simulink model "Gesamtmodell"  (R2017b)
settings: Solver=ode3  StartTime=0.0  StopTime=inf  FixedStep=dt  RelTol=1e-3  EnableMultiTasking=on
InitFcn:
  | Reglerauslegung
undefined symbols (not defined in the file or in its folder): aMax, aMaxPsi, Blindzeit, Com1, dt, K1, K2, K3, Kx, Ky, none, sigbuilder_block, Tx, Ty, vMax, vMaxPsi
libraries: xpcrtudplib x11, simulink x6, xpcutilitieslib x4, xpcseriallib x1, slrtlib x1
(part 3 of 4)

== matlab function Gesamtmodell/Regelung1/Receiver/autoRobID ==
  data: udpIn input; pX output; pY output; psi output; enable output; robID input
function [pX, pY, psi, enable] = autoRobID(udpIn, robID)
enable  = 1;
pX      = 0;
pY      = 0;
psi     = 0;

if robID == 1
    pX      = udpIn(1);
    pY      = udpIn(2);
    psi     = udpIn(3);
elseif robID == 2
    pX      = udpIn(4);
    pY      = udpIn(5);
    psi     = udpIn(6);
elseif robID == 3
    pX      = udpIn(7);
    pY      = udpIn(8);
    psi     = udpIn(9);
elseif robID == 4
    pX      = udpIn(10);
    pY      = udpIn(11);
    psi     = udpIn(12);
elseif robID == 5
    pX      = udpIn(13);
    pY      = udpIn(14);
    psi     = udpIn(15);
end

if (pX == 0) && (pY == 0)
    enable = 0;
end

== matlab function Gesamtmodell/Regelung1/Receiver/x4(psi) ==
  data: psi input; x4 output
function x4 = Winkelkorrektur(psi)

persistent turnCounter firstRun lastAngle

if isempty(firstRun)
    firstRun = 1;
    turnCounter = 0;
    lastAngle = 0;
end

% Kamera gibt uns -pi bis + pi
% Wir wollen 0 bis 2pi
psi = mod(psi+2*pi,2*pi);

% winkel kontinuierlich hoch bzw runterzaehlen
if( (psi < (2*pi)/5) && (lastAngle > ((2*pi) - (2*pi)/5) ) )
    turnCounter = turnCounter + 1;
end

if( (lastAngle < (2*pi)/5) && (psi > ((2*pi) - (2*pi)/5) ) )
    turnCounter = turnCounter - 1;
end

lastAngle = psi;

x4 = psi + turnCounter * 2*pi;

== matlab function Gesamtmodell/Regelung1/Robotino interface/assemble robotino response ==
  data: v_x_in input; robotino_response output; v_y_in input; v_theta_in input; distance_measuring_sensors_in input; bumper_in input; light_barrier_in input; slider_in input
%%%%%%%%%%%%%%%%%%%%%%%%%%%%%%%%%%%%%%%%%%%%%%%%%%%%%%%%%%%%%%%%%%%%%%%%%%%
% Assembly of robot data in a vector of 34 elements.                      %
%                                                                         %
% inputs:   longitudinal, lateral and rotational velocity (in mm/s),      %
%           shaft positions of the three motors (4 elements per motor),   %
%           running times of the three motors (3 elements per motor),     %
%           values of the nine IR-sensors (in mm),                        %
%           bumper collision (1 = no collision;                           %
%                             0 = collision)                              %
% outputs:  vector containing assembled input data                        %
%%%%%%%%%%%%%%%%%%%%%%%%%%%%%%%%%%%%%%%%%%%%%%%%%%%%%%%%%%%%%%%%%%%%%%%%%%%
function robotino_response = fcn(v_x_in, v_y_in, v_theta_in, ...
                                 distance_measuring_sensors_in, ...
                                 bumper_in, light_barrier_in, slider_in)
                                 % motor_positions_in, time_bytes_in, ...)
robotino_response = [light_barrier_in, slider_in, v_x_in, v_y_in, ...
                     v_theta_in, ...%motor_positions_in, time_bytes_in, ...
                     distance_measuring_sensors_in, bumper_in]';

== matlab function Gesamtmodell/Regelung1/Robotino interface/distance converter ==
  settings: sampleTime=dtpc/2
  data: dms_in input; dms_out output
%%%%%%%%%%%%%%%%%%%%%%%%%%%%%%%%%%%%%%%%%%%%%%%%%%%%%%%%%%%%%%%%%%%%%%%%%%%
% conversion of the nine distance measuring sensor values (resolution:    %
% 1Byte) to unit milimeters (range: from 40mm to 1500mm) with linear      %
% interpolation                                                           %
%                                                                         %
% input:  vector containing the values of the nine distance measuring     %
%         sensors                                                         %
% output: vector containing the nine values in milimeters                 %
%%%%%%%%%%%%%%%%%%%%%%%%%%%%%%%%%%%%%%%%%%%%%%%%%%%%%%%%%%%%%%%%%%%%%%%%%%%
function dms_out = fcn(dms_in)

y_mm = [40, 45, 50, 60, 75, 100, 125, 150, 175, 200, 250, 300]; % , ...
        %400, 500, 600, 700, 800, 900, 1000, 1100, 1200, 1300, 1500];
    
x_sensor = [255, 249.7733813, 228.6082474, 193.6871795, ...
            152.0044843, 113.7266187, 92.42268041, ...
            76.36407767, 65.19289827, 55.1025641, ...
            43.06299213, 34.97068404]; % , 24.37410072, ...
            % 16.3381295, 11.62589928, 8.661870504, ...
            % 6.316546763, 4.74, 3.65, 2.96, 2.40, ...
            % 2.035971223, 1.539568345];

% x_sensor = round(100 * x_sensor) / 100;

dms_out = interp1(x_sensor, y_mm, dms_in, 'linear');

== matlab function Gesamtmodell/Regelung1/Robotino interface/light barrier & slider ==
  data: di03_bump_in input; light_barrier output; slider output
function [light_barrier, slider] = fcn(di03_bump_in)
%%%%%%%%%%%%%%%%%%%%%%%%%%%%%%%%%%%%%%%%%%%%%%%%%%%%%%%%%%%%%%%%%%%%%%%%%%%
% di03_bump_in = 0 alternatively 12 ->  no light barrier activation       %
%                                       no slider activation              %
% di03_bump_in = 13                 ->  only light barrier activation     %
% di03_bump_in = 14                 ->  only slider activation            %
% di03_bump_in = 15                 ->  light barrier activation          %
%                                       slider activation                 %
%%%%%%%%%%%%%%%%%%%%%%%%%%%%%%%%%%%%%%%%%%%%%%%%%%%%%%%%%%%%%%%%%%%%%%%%%%%
% function [light_barrier, slider] = fcn(di03_bump_in)
% bin = dec2bin(di03_bump_in);
% if bin(3) == 1
%     light_barrier = 1;
% else
%     light_barrier = 0;
% end
% if bin(4) == 1
%     slider = 1;
% else
%     slider = 0;
% end
if     di03_bump_in == 13
    light_barrier = 1;
    slider        = 0;
elseif di03_bump_in == 14
    light_barrier = 0;
    slider        = 1;
elseif di03_bump_in == 15
    light_barrier = 1;
    slider        = 1;
else
    light_barrier = 0;
    slider        = 0;
end

== matlab function Gesamtmodell/Regelung1/Robotino interface/receive direction, unit & velocity converter ==
  settings: sampleTime=dtpc/2
  data: number_of_robot input; direction_motor0_in input; v_x_out output; velocity_motor0_in input; direction_motor1_in input; velocity_motor1_in input; direction_motor2_in input; velocity_motor2_in input; v_y_out output; v_theta_out output
%%%%%%%%%%%%%%%%%%%%%%%%%%%%%%%%%%%%%%%%%%%%%%%%%%%%%%%%%%%%%%%%%%%%%%%%%%%
% assembly of the three separate positive motor velocities (resolution:   %
% 1Byte) and their rotation direction to positive and/or negative         %
% longitudinal, lateral & rotational velocities (in milimeters per        %
% second)                                                                 %
%                                                                         %
% inputs:  direction_motor0_in (rotating direction of motor0              %
%          (129 := counter-clockwise; 128 := clockwise)),                 %
%          velocity_motor0_in (from 0 to 255),                            %
%          direction_motor1_in (rotating direction of motor1              %
%          (0 := counter-clockwise; 1 := clockwise)),                     %
%          velocity_motor1_in (from 0 to 255),                            %
%          direction_motor2_in (rotating direction of motor2              %
%          (0 := counter-clockwise; 1 := clockwise)),                     %
%          velocity_motor2_in (from 0 to 255)                             %
% outputs: v_x_out (longitudinal velocity (in milimeters per second)),    %
%          v_y_out (lateral velocity (in milimeters per second)),         %
%          v_theta_out (rotational velocity (in milimeters per second))   %
%%%%%%%%%%%%%%%%%%%%%%%%%%%%%%%%%%%%%%%%%%%%%%%%%%%%%%%%%%%%%%%%%%%%%%%%%%%
function [v_x_out, v_y_out, v_theta_out] ...
    = fcn(number_of_robot, direction_motor0_in, velocity_motor0_in, direction_motor1_in, ...
          velocity_motor1_in, direction_motor2_in, velocity_motor2_in)
%%%%%%%%%%%%%%%%%%%%%%%%%%%%%%%%%%%%%%%%%%%%%%%%%%%%%%%%%%%%%%%%%
% assembly of absolute motor velocity and rotating direction to %
% longitudinal, lateral & rotational velocity for every motor   %
%%%%%%%%%%%%%%%%%%%%%%%%%%%%%%%%%%%%%%%%%%%%%%%%%%%%%%%%%%%%%%%%%


% the direction bit for the motor 0 of robotino 3 is located at a different position
if number_of_robot == 3
    cmp = 1;
else
    cmp = 129;
end
    

if direction_motor0_in < cmp
    v0 = -velocity_motor0_in;
else
    v0 =  velocity_motor0_in;
end

if direction_motor1_in < 1
    v1 = -velocity_motor1_in;
else
    v1 =  velocity_motor1_in;
end

if direction_motor2_in < 1
    v2 = -velocity_motor2_in;
else
    v2 =  velocity_motor2_in;
end

%%%%%%%%%%%%%%%%%%%%%%%%%%%%%%%%%%%%%%%%%%%%%%%%%%%%%%%%%%%%%%%%%%%%%%%%%
% conversion of the separate motor velocities from a value between -255 %
% and 255 to millimeters                                                %
%%%%%%%%%%%%%%%%%%%%%%%%%%%%%%%%%%%%%%%%%%%%%%%%%%%%%%%%%%%%%%%%%%%%%%%%%
f_rcv = 7.02;
v0    = v0 * f_rcv;
v1    = v1 * f_rcv;
v2    = v2 * f_rcv;

%%%%%%%%%%%%%%%%%%%%%%%%%%%%%%%%%%%%%%%%%%%%%%%%%%%%%%%%%%%%%%%%%%%%
% conversion from three separate motor velocities to longitudinal, %
% lateral & rotational velocity                                    %
%%%%%%%%%%%%%%%%%%%%%%%%%%%%%%%%%%%%%%%%%%%%%%%%%%%%%%%%%%%%%%%%%%%%
v_x_out     = (v2 - v0) / (2 * cosd(30));                         % in mm/s
v_y_out     = (v0 - 2 * v1 + v2) / 3;                             % in mm/s
v_theta_out = (v0 + v1 + v2) / (3 * 135);                        % in rad/s

== matlab function Gesamtmodell/Regelung1/Robotino interface/serial communication/error filter & protocol disassembler ==
  settings: sampleTime=dtpc/2
  data: response input; error_free_resp_in input; direction_motor0_out output; velocity_motor0_out output; direction_motor1_out output; velocity_motor1_out output; direction_motor2_out output; velocity_motor2_out output; distance_measuring_sensors_out output; di03_bump_out output; bumper_out output; error_free_resp_out output
%%%%%%%%%%%%%%%%%%%%%%%%%%%%%%%%%%%%%%%%%%%%%%%%%%%%%%%%%%%%%%%%%%%%%%%%%%%
% Error check of the 'I/O-Board to PC104 message' and filtering of this   %
% defective response: Substitute defective message by the last error free %
% message.                                                                %
% Saving of the rotating direction, velocity, shaft position and running  %
% time of the three motors. Combining all shaft positions in a vector.    %
% Combining all running times in a vector.                                %
% Saving of the three bumper bytes indicating a collision in a vector.    %
% Saving the values of the nine distance measuring IR-sensors in a vector.%
%                                                                         %
% inputs: response (actual 'I/O-Board to PC104 message')(vector 102       %
%                   elements)                                             %
%         error_free_resp_in (last error free 'I/O-Board to PC104         %
%                             message')                                   %
% outputs: directions and velocities of the three motors                  %
%          motor_positions_out (shaft positions of the three motors)      %
%                              (vector 12 elements)                       %
%          time_bytes_out (running times of the three motors)             %
%                         (vector 9 elements)                             %
%          distance_measuring_sensors_out (values of the nine IR-sensors) %
%                                         (vector 9 elements)             %
%          bumper_out (vector 3 elements)                                 %
%          error_free_resp_out (error free 'I/O-Board to PC104 message')  %
%                              (vector 102 elements)                      %
%%%%%%%%%%%%%%%%%%%%%%%%%%%%%%%%%%%%%%%%%%%%%%%%%%%%%%%%%%%%%%%%%%%%%%%%%%%
function [direction_motor0_out, velocity_motor0_out, ...
          direction_motor1_out, velocity_motor1_out, ...
          direction_motor2_out, velocity_motor2_out, ...
          distance_measuring_sensors_out, di03_bump_out, bumper_out, ...
          error_free_resp_out] = fcn(response, error_free_resp_in)
%           motor_positions_out, time_bytes_out, ...)
      
%%%%%%%%%%%%%%%%%%%%%%%%%%%%%%%%%%%%%%%%%%%%%%%%%%%%%
% filtering defective 'I/O-Board to PC104 messages' %
%%%%%%%%%%%%%%%%%%%%%%%%%%%%%%%%%%%%%%%%%%%%%%%%%%%%%
if (response(1) == 101) && (response(2) == 82) && (response(3) == 69) ...
   && (response(4) == 67) && (response(100) == 114) ...        % if the ...
   && (response(101) == 101) && (response(102) == 99)  % counter (101), ...
                        % the start (REC) and stop (rec) bytes are true ...
    error_free_resp_out = response;     % save the actual 'I/O-Board to ...
                                                           % PC104 message'
else                                                        % otherwise ...
    error_free_resp_out = error_free_resp_in;     % save the last error ...
                                        % free 'I/O-Board to PC104 message'
end

%%%%%%%%%%%%%%%%%%%%%%%%%%%%%%%%%%%%%%%%%%%%%%%%%%%%%%%%%%%%%%%%%%%%%%%%%%
% save rotating direction, velocity, shaft position and the running time %
% of motor0                                                              %
%%%%%%%%%%%%%%%%%%%%%%%%%%%%%%%%%%%%%%%%%%%%%%%%%%%%%%%%%%%%%%%%%%%%%%%%%%
direction_motor0_out  = error_free_resp_out(26);
velocity_motor0_out   = error_free_resp_out(27);
% position_motor0_byte1 = error_free_resp_out(28);
% position_motor0_byte2 = error_free_resp_out(29);
% position_motor0_byte3 = error_free_resp_out(30);
% position_motor0_byte4 = error_free_resp_out(31);
% time_motor0_byte1     = error_free_resp_out(34);
% time_motor0_byte2     = error_free_resp_out(35);
% time_motor0_byte3     = error_free_resp_out(36);

%%%%%%%%%%%%%%%%%%%%%%%%%%%%%%%%%%%%%%%%%%%%%%%%%%%%%%%%%%%%%%%%%%%%%%%%%%
% save rotating direction, velocity, shaft position and the running time %
% of motor1                                                              %
%%%%%%%%%%%%%%%%%%%%%%%%%%%%%%%%%%%%%%%%%%%%%%%%%%%%%%%%%%%%%%%%%%%%%%%%%%
direction_motor1_out  = error_free_resp_out(47);
velocity_motor1_out   = error_free_resp_out(48);
% position_motor1_byte1 = error_free_resp_out(49);
% position_motor1_byte2 = error_free_resp_out(50);
% position_motor1_byte3 = error_free_resp_out(51);
% position_motor1_byte4 = error_free_resp_out(52);
% time_motor1_byte1     = error_free_resp_out(55);
% time_motor1_byte2     = error_free_resp_out(56);
% time_motor1_byte3     = error_free_resp_out(57);

%%%%%%%%%%%%%%%%%%%%%%%%%%%%%%%%%%%%%%%%%%%%%%%%%%%%%%%%%%%%%%%%%%%%%%%%%%
% save rotating direction, velocity, shaft position and the running time %
% of motor2                                                              %
%%%%%%%%%%%%%%%%%%%%%%%%%%%%%%%%%%%%%%%%%%%%%%%%%%%%%%%%%%%%%%%%%%%%%%%%%%
direction_motor2_out  = error_free_resp_out(68);
velocity_motor2_out   = error_free_resp_out(69);
% position_motor2_byte1 = error_free_resp_out(70);
% position_motor2_byte2 = error_free_resp_out(71);
% position_motor2_byte3 = error_free_resp_out(72);
% position_motor2_byte4 = error_free_resp_out(73);
% time_motor2_byte1     = error_free_resp_out(76);
% time_motor2_byte2     = error_free_resp_out(77);
% time_motor2_byte3     = error_free_resp_out(78);

%%%%%%%%%%%%%%%%%%%%%%%%%%%%%%%%%%%%%%%%%%%
% save the three bumper bytes in a vector %
%%%%%%%%%%%%%%%%%%%%%%%%%%%%%%%%%%%%%%%%%%%
bumper_out = [error_free_resp_out(32), error_free_resp_out(53), ...
              error_free_resp_out(74)]';
          
%%%%%%%%%%%%%%%%%%%%%%%%%%%%%%%%%%%%%%%%%%%%%%%%%%%%%%%%%%%%%%%%%%%%%%
% save the values of the nine distance measuring sensors in a vector %
%%%%%%%%%%%%%%%%%%%%%%%%%%%%%%%%%%%%%%%%%%%%%%%%%%%%%%%%%%%%%%%%%%%%%%
distance_measuring_sensors_out = [error_free_resp_out(60), ...
                    error_free_resp_out(59), error_free_resp_out(44), ...
                    error_free_resp_out(39), error_free_resp_out(38), ...
                    error_free_resp_out(17), error_free_resp_out(18), ...
                    error_free_resp_out(23), error_free_resp_out(65)];
                
%%%%%%%%%%%%%%%%%%%%%%%%%%%%%%%%%%%%%%%%%%%%%%%%%%%%%%%%
% save positions of the three motor shafts in a vector %
%%%%%%%%%%%%%%%%%%%%%%%%%%%%%%%%%%%%%%%%%%%%%%%%%%%%%%%%
% motor_positions_out = [position_motor0_byte1, position_motor0_byte2, ...
%                        position_motor0_byte3, position_motor0_byte4, ...
%                        position_motor1_byte1, position_motor1_byte2, ...
%                        position_motor1_byte3, position_motor1_byte4, ...
%                        position_motor2_byte1, position_motor2_byte2, ...
%                        position_motor2_byte3, position_motor2_byte4];

%%%%%%%%%%%%%%%%%%%%%%%%%%%%%%%%%%%%%%%%%%%%%%%%%%%%%%%%%%
% save the running times of the three motors in a vector %
%%%%%%%%%%%%%%%%%%%%%%%%%%%%%%%%%%%%%%%%%%%%%%%%%%%%%%%%%%
% time_bytes_out = [time_motor0_byte1, time_motor0_byte2, ...
%                   time_motor0_byte3, time_motor1_byte1, ...
%                   time_motor1_byte2, time_motor1_byte3, ...
%                   time_motor2_byte1, time_motor2_byte2, time_motor2_byte3];

%%%%%%%%%%%%%%%%%%%%%%%%%%%%%%%%%%%%%%
% save values of digital input 0 - 3 %
%%%%%%%%%%%%%%%%%%%%%%%%%%%%%%%%%%%%%%
di03_bump_out = error_free_resp_out(32);

== matlab function Gesamtmodell/Regelung1/Robotino interface/serial communication/protocol adder & optional velocity adaption ==
  settings: sampleTime=2*dtpc
  data: dir input; vel input; direction_motor0_in input; velocity_motor0_in input; direction_motor1_in input; velocity_motor1_in input; direction_motor2_in input; velocity_motor2_in input; stop_in input; message output
%%%%%%%%%%%%%%%%%%%%%%%%%%%%%%%%%%%%%%%%%%%%%%%%%%%%%%%%%%%%%%%%%%%%%%%%%%%
% parameterising the 'PC104 to I/O-Board message' for serial line         %
% communication with control commands for the robotino motors             %
%                                                                         %
% optional: velocity adaption as soon as at least one motor is near the   %
%           speed limit                                                   %
%                                                                         %
% inputs: rotating directions and velocities of the three motors          %
% output: vector containing the 'PC104 to I/O-Board message' for serial   %
%         line communication                                              %
%%%%%%%%%%%%%%%%%%%%%%%%%%%%%%%%%%%%%%%%%%%%%%%%%%%%%%%%%%%%%%%%%%%%%%%%%%%
function message = fcn(dir, vel, direction_motor0_in, velocity_motor0_in, ...
                       direction_motor1_in, velocity_motor1_in, ...
                       direction_motor2_in, velocity_motor2_in, stop_in)
%%%%%%%%%%%%%%%%%%%%%%%%%%%%%%
% optional velocity adaption %
%%%%%%%%%%%%%%%%%%%%%%%%%%%%%%
vmax = 175;                                               % v_motor_dez_max

if velocity_motor0_in > vmax
    velocity_motor0_tf = velocity_motor0_in;
    
    velocity_motor0_in = vmax;
    velocity_motor1_in = vmax * velocity_motor1_in / velocity_motor0_tf;
    velocity_motor2_in = vmax * velocity_motor2_in / velocity_motor0_tf;
end

if velocity_motor1_in > vmax
    velocity_motor1_tf = velocity_motor1_in;
    
    velocity_motor0_in = vmax * velocity_motor0_in / velocity_motor1_tf;
    velocity_motor1_in = vmax;
    velocity_motor2_in = vmax * velocity_motor2_in / velocity_motor1_tf;
end

if velocity_motor2_in > vmax
    velocity_motor2_tf = velocity_motor2_in;
    
    velocity_motor0_in = vmax * velocity_motor0_in / velocity_motor2_tf;
    velocity_motor1_in = vmax * velocity_motor1_in / velocity_motor2_tf;
    velocity_motor2_in = vmax;
end
%%%%%%%%%%%%%%%%%%%%%%%%%%%%%%%%%%%%%%%%%%%%%%%%%%%%%%%%%%%%%%%%%%%%%%
% vector containing the 'PC104 to I/O-Board message' for serial line %
% communication                                                      %
%%%%%%%%%%%%%%%%%%%%%%%%%%%%%%%%%%%%%%%%%%%%%%%%%%%%%%%%%%%%%%%%%%%%%%
message = [47, abs('REC'), 5, min(stop_in), direction_motor0_in, ...
           velocity_motor0_in, zeros(1, 4), 255, 255, 255, ...
           min(stop_in), direction_motor1_in, velocity_motor1_in, ...
           zeros(1, 4), 255, 255, 255, min(stop_in), ...
           direction_motor2_in, velocity_motor2_in, zeros(1, 4), 255, ...
           255, 255, 1, dir, vel, zeros(1, 4), 255, 255, 255, abs('rec')].';

== matlab function Gesamtmodell/Regelung1/Robotino interface/serial communication/stop by bumper ==
  settings: sampleTime=2*dtpc
  data: stop_out output; bumper input; stop_flag_in input; stop_flag_out output
%%%%%%%%%%%%%%%%%%%%%%%%%%%%%%%%%%%%%%%%%%%%%%%%%%%%%%%%%%%%%%%%%%%%%%%%%%%
% Recognition of collisions and creating of variables indicating and      %
% marking a collision                                                     %
%                                                                         %
% inputs: bumper (vector of the three bumper bytes)                       %
%         stop_flag_in (As long as no collision has occured,              %
%                       'stop_flag_in' contains the last bumper vector    %
%                       indicating no collision.                          %
%                       If a collision has occured, 'stop_flag_in'        %
%                       contains the last bumper vector indicating a      %
%                       collision until the simulation stops.)            %
% outputs: stop_out (indicates a collision: 1 = no collision;             %
%                                           0 = collision)                %
%          stop_flag_out (gets the actual bumper vector unless 'bumper'   %
%                         indicates no collision and 'stop_flag_in'       %
%                         indicates a past collision.)                    %
%%%%%%%%%%%%%%%%%%%%%%%%%%%%%%%%%%%%%%%%%%%%%%%%%%%%%%%%%%%%%%%%%%%%%%%%%%%
function [stop_out, stop_flag_out] = fcn(bumper, stop_flag_in)
if max(bumper) == 31       % as soon as the maximum value of the bumper ...
                              % vector indicates 31 a collision is detected
    stop_out = 0;
    stop_flag_out = bumper;
elseif max(stop_flag_in) == 31 % if the maximum value of 'stop_flag_in' ...
                                      % indicates a past collision (31) ...
    stop_out = 0;         % 'stop_out' gets 0 for a further stop of the ...
                                                           % motors and ...
    stop_flag_out = stop_flag_in; % 'stop_flag_out' gets the last bumper...
                                       % vector indicating a past collision
else                                                        % otherwise ...
    stop_out = 1;    % 'stop_out' gets 1 to keep the motors running and ...
    stop_flag_out = bumper; % 'stop_flag_out' gets the actual bumper vector
end

== matlab function Gesamtmodell/Regelung1/Robotino interface/transmit velocity, unit & direction converter ==
  settings: sampleTime=2*dtpc
  data: direction_motor0_out output; velocity_motor0_out output; direction_motor1_out output; velocity_motor1_out output; direction_motor2_out output; velocity_motor2_out output; v_x_in input; v_y_in input; v_theta_in input
%%%%%%%%%%%%%%%%%%%%%%%%%%%%%%%%%%%%%%%%%%%%%%%%%%%%%%%%%%%%%%%%%%%%%%%%%%%
% conversion from positive and/or negative longitudinal, lateral and      %
% rotational velocities (in milimeters per second) to three separate      %
% positive motor velocities (resolution: 1Byte) and their rotation        %
% direction                                                               %
%                                                                         %
% inputs:  v_x_in (longitudinal velocity in milimeters per second),       %
%          v_y_in (lateral velocity in milimeters per second),            %
%          v_theta_in (rotational velocity in milimeters per second)      %
% outputs: direction_motor0_out (rotating direction of motor0             %
%          (0 := counter-clockwise; 2 := clockwise)),                     %
%          velocity_motor0_out (from 0 to 255),                           %
%          direction_motor1_out (rotating direction of motor1             %
%          (0 := counter-clockwise; 2 := clockwise)),                     %
%          velocity_motor1_out (from 0 to 255),                           %
%          direction_motor2_out (rotating direction of motor2             %
%          (0 := counter-clockwise; 2 := clockwise)),                     %
%          velocity_motor2_out (from 0 to 255)                            %
%%%%%%%%%%%%%%%%%%%%%%%%%%%%%%%%%%%%%%%%%%%%%%%%%%%%%%%%%%%%%%%%%%%%%%%%%%%
function [direction_motor0_out, velocity_motor0_out, ...
          direction_motor1_out, velocity_motor1_out, ...
          direction_motor2_out, velocity_motor2_out] ...
                                          = fcn(v_x_in, v_y_in, v_theta_in)
%%%%%%%%%%%%%%%%%%%%%%%%%%%%%%%%%%%%%%%%%%%%%%%%%%%%%%%%%%%%%%%%%%%%%%
% conversion from longitudinal, lateral & rotational velocity to the %
% three separate motor velocities                                    %
%%%%%%%%%%%%%%%%%%%%%%%%%%%%%%%%%%%%%%%%%%%%%%%%%%%%%%%%%%%%%%%%%%%%%%
v0 = (-v_x_in * cosd(30)) + ( v_y_in * cosd(60)) + (v_theta_in * 135);
v1 =                      + (-v_y_in)            + (v_theta_in * 135);
v2 = ( v_x_in * cosd(30)) + ( v_y_in * cosd(60)) + (v_theta_in * 135);

%%%%%%%%%%%%%%%%%%%%%%%%%%%%%%%%%%%%%%%%%%%%%%%%%%%%%%%%%%%%%%%%%%%%%
% conversion of the separate motor velocities from millimeters to a %
% value between -255 and 255                                        %
%%%%%%%%%%%%%%%%%%%%%%%%%%%%%%%%%%%%%%%%%%%%%%%%%%%%%%%%%%%%%%%%%%%%%
f = 1 / 7.02;
v0 = v0 * f;
v1 = v1 * f;
v2 = v2 * f;

%%%%%%%%%%%%%%%%%%%%%%%%%%%%%%%%%%%%%%%%%%%%%%%%%%%%%%%%%%%%%%%%%%%%
% division of motor velocities into absolute velocity and rotating %
% direction                                                        %
%%%%%%%%%%%%%%%%%%%%%%%%%%%%%%%%%%%%%%%%%%%%%%%%%%%%%%%%%%%%%%%%%%%%
if v0 < 0
    direction_motor0_out =  0;
    velocity_motor0_out  = -v0;
else
    direction_motor0_out = 2;
    velocity_motor0_out  = v0;
end

if v1 < 0
    direction_motor1_out =  0;
    velocity_motor1_out  = -v1;
else
    direction_motor1_out = 2;
    velocity_motor1_out  = v1;
end

if v2 < 0
    direction_motor2_out =  0;
    velocity_motor2_out  = -v2;
else
    direction_motor2_out = 2;
    velocity_motor2_out  = v2;
end

== matlab function Gesamtmodell/Regelung1/Stellgrößen- beschränkung /Beschraenkung  ==
  data: MaxStellT input; MaxStellR input; x input; X output; Y output; y input; theta input; Theta output
function [X,Y,Theta] = Beschraenkung(MaxStellT,MaxStellR,x,y,theta)

if (x > MaxStellT)
    X = MaxStellT;
elseif  (x < -MaxStellT)
    X = -MaxStellT;
else 
    X = x;
end

if (y > MaxStellT)
    Y = MaxStellT;
elseif  (y < -MaxStellT)
    Y = -MaxStellT;
else
    Y = y;
end

if (theta > MaxStellR)
    Theta = MaxStellR;
elseif  (theta < -MaxStellR)
    Theta = -MaxStellR;
else
    Theta = theta;
end

== matlab function Gesamtmodell/Regelung1/Zustandsautomat/Bahnplanung Psi ==
  settings: updateMethod=DISCRETE  sampleTime=dt
  data: zielPosition input; istPosition input; enable input; sollPosition output; dt parameter; sollGeschwindigkeit output; aMaxPsi parameter; vMaxPsi parameter
% s = 1/2 * m * t^2
% v = m * t
% a = m

function [sollPosition, sollGeschwindigkeit]= Bahnplanung(zielPosition,istPosition,enable,dt,aMaxPsi,vMaxPsi)
    
%     aMax = 0.5;  % Maximale Beschleunigung
%     vMax = 2; % Maximale Geschwindigkeit
     nGr = 1000; % Groesse der Planvektoren

    persistent firstRun s v nZyklen nZyklenK fertig  n
    
    if isempty(firstRun)
        firstRun = 1;
        s = 0;          % Vektor mit Wegdaten
        v = 0;          % Vektor mit Geschwindigkeitsdaten
        nZyklen = 0;    % Anzahl der benoetigten Zyklen
        nZyklenK = 0;
        n = 1;          % Zaehlvariable
        fertig = 0;
    end

    if (enable == 1) || (fertig == 1)
        n = 1;
        Out = 1;
        startPosition = mod(istPosition,2*pi);
        % Berechnung der optimalen Drehrichtung
        
        if (abs(zielPosition-startPosition) <= pi)   % (1)
    
            Out = zielPosition - startPosition;      % (2)

        else

             if (zielPosition > startPosition)                % (3)
                Out = zielPosition - startPosition - 2*pi;    % (4)
             else
                 Out = zielPosition - startPosition + 2*pi;   % (5)
             end
        end
        
        % Berechnung der Zeitabschnitte für anfahren, konstant Fahren und bremsen
        tvMax   = 1/aMaxPsi * vMaxPsi ;       % Zeit bis maximale Geschw.(vMax) erreicht ist
        svMax   = 1/2 * aMaxPsi * tvMax^2; % Weg der zurueckgelegt wurde bis tvMax
        tK      = (abs(Out) - 2 * svMax) / vMaxPsi; % Zeit waehrend konstant gefahren wird
        % Fuer nur Anfahren und Bremsen
        tHalbe = sqrt(2 * 1/aMaxPsi * abs(Out)/2); % Zeit bis zur halben Strecke

        tBB = zeros(1,nGr);
        tBA = zeros(1,nGr);
        tBK = zeros(1,nGr);
        sA  = zeros(1,nGr);
        vA  = zeros(1,nGr);
        sB  = zeros(1,nGr);
        vB  = zeros(1,nGr);
        sK  = zeros(1,nGr);
        vK  = zeros(1,nGr);
        s   = zeros(1,3*nGr);
        v   = zeros(1,3*nGr);
        
        
        % Nur Anfahren und Bremsen
         if tvMax > tHalbe
            % Beschleunigung/Anfahrt
            nZyklen = ceil(tHalbe/dt);
            nZyklenK = 0;
            if nZyklen > nGr
                nZyklen = nGr;
            elseif nZyklen <= 0
                nZyklen = 1;
            end
            
            tBA(1:nZyklen) = linspace(0,tHalbe,nZyklen);%0:dt:(nZyklen)*dt-dt;

            sA(1:nZyklen) = sign(Out) * 1/2 * aMaxPsi * tBA(1:nZyklen).^2;
            vA(1:nZyklen) = sign(Out) *aMaxPsi * tBA(1:nZyklen);
            if sA(nZyklen) == 0
                offset = 1;
            else
                offset = 0;
            end
            % Bremsen
            tBB(1:nZyklen) = linspace(-tHalbe,0,nZyklen);%-nZyklen*dt+dt:dt:0;

            sB(1:nZyklen) = -sign(Out) * 1/2 * aMaxPsi * tBB(1:nZyklen) .^2 + 2*sA(nZyklen-offset);
            vB(1:nZyklen) = -sign(Out) * aMaxPsi * tBB(1:nZyklen);
            s(1:2*nZyklen) = [sA(1:nZyklen) sB(1:nZyklen)]+startPosition;
            v(1:2*nZyklen) = [vA(1:nZyklen) vB(1:nZyklen)];
            
        else
            % Beschleunigung/Anfahrt

            nZyklen = ceil((tvMax)/dt);
            nZyklenK = ceil(tK/dt);

            if nZyklen > nGr
                nZyklen = nGr;
            elseif nZyklen <= 0
                nZyklen = 1;
            end
            if nZyklenK > nGr
                nZyklenK = nGr;
            elseif nZyklenK <= 0
                nZyklenK = 1;
            end
            
            tBA(1:nZyklen) = linspace(0,tvMax,nZyklen);%0:dt:(nZyklen)*dt-dt;

            sA(1:nZyklen) = sign(Out) * 1/2 * aMaxPsi * tBA(1:nZyklen).^2;
            vA(1:nZyklen) = sign(Out) * aMaxPsi * tBA(1:nZyklen);
            if sA(nZyklen) == 0
                offset = 1;
            else
                offset = 0;
            end
            % Fahrt mit konstanter Geschwindigkeit
            tBK(1:nZyklenK) = linspace(0,tK,nZyklenK);%0:dt:(nZyklenK)*dt-dt;
            vK(1:nZyklenK)   = sign(Out) * vMaxPsi * ones(1,nZyklenK);
            sK(1:nZyklenK)   = sign(Out) * vMaxPsi * tBK(1:nZyklenK) + sA(nZyklen-offset);
            if sK(nZyklenK) == 0
                offsetK = 1;
            else
                offsetK = 0;
            end
            % Bremsen
            tBB(1:nZyklen) = linspace(-tvMax,0,nZyklen);%-(nZyklen)*dt+dt:dt:0;

            sB(1:nZyklen) = -sign(Out) *  1/2 * aMaxPsi * tBB(1:nZyklen).^2 + sA(nZyklen-offset)+sK(nZyklenK-offsetK);
            vB(1:nZyklen) = -sign(Out) *  aMaxPsi * tBB(1:nZyklen);
            s(1:2*nZyklen+nZyklenK) = [sA(1:nZyklen) sK(1:nZyklenK) sB(1:nZyklen)]+startPosition;
            v(1:2*nZyklen+nZyklenK) = [vA(1:nZyklen) vK(1:nZyklenK) vB(1:nZyklen)];
         end
        firstRun = 0;
    end
    % Ausgabe
    sollPosition = s(n);
    sollGeschwindigkeit = v(n);
    if n < (2*nZyklen+nZyklenK-1)
        n = n + 1;
         fertig = 0;
     elseif nZyklen == nGr || nZyklenK == nGr 
         fertig = 1;
    end

== matlab function Gesamtmodell/Regelung1/Zustandsautomat/Bahnplanung X ==
  settings: updateMethod=DISCRETE  sampleTime=dt
  data: zielPosition input; istPosition input; enable input; sollPosition output; dt parameter; sollGeschwindigkeit output; aMax parameter; vMax parameter
% s = 1/2 * m * t^2
% v = m * t
% a = m

function [sollPosition, sollGeschwindigkeit]= Bahnplanung(zielPosition,istPosition,enable,dt,aMax,vMax)
    
%     aMax = 300;  % Maximale Beschleunigung
%     vMax = 500; % Maximale Geschwindigkeit
     nGr = 1000; % Groesse der Planvektoren

    persistent firstRun s v nZyklen nZyklenK fertig  n
    
    if isempty(firstRun)
        firstRun = 1;
        s = 0;          % Vektor mit Wegdaten
        v = 0;          % Vektor mit Geschwindigkeitsdaten
        nZyklen = 0;    % Anzahl der benoetigten Zyklen
        nZyklenK = 0;
        n = 1;          % Zaehlvariable
        fertig = 0;
    end

    if (enable == 1) || (fertig == 1)
        n = 1;
        startPosition = istPosition;
        % Berechnung der Zeitabschnitte für anfahren, konstant Fahren und bremsen
        tvMax   = 1/aMax * vMax ;       % Zeit bis maximale Geschw.(vMax) erreicht ist
        svMax   = 1/2 * aMax * tvMax^2; % Weg der zurueckgelegt wurde bis tvMax
        tK      = (abs(zielPosition-startPosition) - 2 * svMax) / vMax; % Zeit waehrend konstant gefahren wird
        % Fuer nur Anfahren und Bremsen
        tHalbe = sqrt(2 * 1/aMax * abs(zielPosition-startPosition)/2); % Zeit bis zur halben Strecke

        tBB = zeros(1,nGr);
        tBA = zeros(1,nGr);
        tBK = zeros(1,nGr);
        sA  = zeros(1,nGr);
        vA  = zeros(1,nGr);
        sB  = zeros(1,nGr);
        vB  = zeros(1,nGr);
        sK  = zeros(1,nGr);
        vK  = zeros(1,nGr);
        s   = zeros(1,3*nGr);
        v   = zeros(1,3*nGr);
%         % Nur Anfahren und Bremsen
         if tvMax > tHalbe
            % Beschleunigung/Anfahrt
            nZyklen = ceil(tHalbe/dt);
            nZyklenK = 0;
            if nZyklen > nGr
                nZyklen = nGr;
            elseif nZyklen <= 0
                nZyklen = 1;
            end
            
            tBA(1:nZyklen) = linspace(0,tHalbe,nZyklen);%0:dt:(nZyklen)*dt-dt;

            sA(1:nZyklen) = sign(zielPosition-startPosition) * 1/2 * aMax * tBA(1:nZyklen).^2;
            %sA(sA==0) = [];
            vA(1:nZyklen) = sign(zielPosition-startPosition) *aMax * tBA(1:nZyklen);
            % Bremsen
            tBB(1:nZyklen) = linspace(-tHalbe,0,nZyklen);%-nZyklen*dt+dt:dt:0;
            
            %manchmal klappt das mit dem runden nicht so gut...
            if sA(nZyklen) == 0
                offset = 1;
            else
                offset = 0;
            end
            
            sB(1:nZyklen) = -sign(zielPosition-startPosition) * 1/2 * aMax * tBB(1:nZyklen) .^2 + 2*sA(nZyklen-offset);
            vB(1:nZyklen) = -sign(zielPosition-startPosition) * aMax * tBB(1:nZyklen);
            s(1:2*nZyklen) = [sA(1:nZyklen) sB(1:nZyklen)]+startPosition;
            v(1:2*nZyklen) = [vA(1:nZyklen) vB(1:nZyklen)];
            
        else
            % Beschleunigung/Anfahrt

            nZyklen = ceil((tvMax)/dt);
            nZyklenK = ceil(tK/dt);

            if nZyklen > nGr
                nZyklen = nGr;
            elseif nZyklen <= 0
                nZyklen = 1;
            end
            if nZyklenK > nGr
                nZyklenK = nGr;
            elseif nZyklenK <= 0
                nZyklenK = 1;
            end
            
            tBA(1:nZyklen) = linspace(0,tvMax,nZyklen);%0:dt:(nZyklen)*dt-dt;

            sA(1:nZyklen) = sign(zielPosition-startPosition) * 1/2 * aMax * tBA(1:nZyklen).^2;
            vA(1:nZyklen) = sign(zielPosition-startPosition) * aMax * tBA(1:nZyklen);
            %manchmal klappt das mit dem runden nicht so gut...
            if sA(nZyklen) == 0
                offset = 1;
            else
                offset = 0;
            end
            % Fahrt mit konstanter Geschwindigkeit
            tBK(1:nZyklenK) = linspace(0,tK,nZyklenK);%0:dt:(nZyklenK)*dt-dt;
            vK(1:nZyklenK)   = sign(zielPosition-startPosition) * vMax * ones(1,nZyklenK);
            
            % wieso wir hier im gegensatz zu sB nur einmal sA
            % draufgerechnet statt 2*sA ?
            sK(1:nZyklenK)   = sign(zielPosition-startPosition) * vMax * tBK(1:nZyklenK) + sA(nZyklen-offset);
            
            if sK(nZyklenK) == 0
                offsetK = 1;
            else
                offsetK = 0;
            end
            % Bremsen
            tBB(1:nZyklen) = linspace(-tvMax,0,nZyklen);%-(nZyklen)*dt+dt:dt:0;
            %sB(1:nZyklen) = -sign(zielPosition-startPosition) * 1/2 * aMax * tBB(1:nZyklen) .^2 + 2*sA(nZyklen-offset);
            sB(1:nZyklen) = -sign(zielPosition-startPosition) *  1/2 * aMax * tBB(1:nZyklen).^2 + sA(nZyklen-offset)+sK(nZyklenK-offsetK);
            vB(1:nZyklen) = -sign(zielPosition-startPosition) *  aMax * tBB(1:nZyklen);
            s(1:2*nZyklen+nZyklenK) = [sA(1:nZyklen) sK(1:nZyklenK) sB(1:nZyklen)]+startPosition;
            v(1:2*nZyklen+nZyklenK) = [vA(1:nZyklen) vK(1:nZyklenK) vB(1:nZyklen)];
         end
        firstRun = 0;
    end
    % Ausgabe
    sollPosition = s(n);
    sollGeschwindigkeit = v(n);
    if n < (2*nZyklen+nZyklenK-1)
        n = n + 1;
         fertig = 0;
     elseif nZyklen == nGr || nZyklenK == nGr 
         fertig = 1;
    end

== matlab function Gesamtmodell/Regelung1/Zustandsautomat/Bahnplanung Y ==
  settings: updateMethod=DISCRETE  sampleTime=dt
  data: zielPosition input; istPosition input; enable input; sollPosition output; dt parameter; sollGeschwindigkeit output; aMax parameter; vMax parameter
% s = 1/2 * m * t^2
% v = m * t
% a = m

function [sollPosition, sollGeschwindigkeit]= Bahnplanung(zielPosition,istPosition,enable,dt,aMax,vMax)
    
%     aMax = 300;  % Maximale Beschleunigung
%     vMax = 500; % Maximale Geschwindigkeit
     nGr = 1000; % Groesse der Planvektoren

    persistent firstRun s v nZyklen nZyklenK fertig  n
    
    if isempty(firstRun)
        firstRun = 1;
        s = 0;          % Vektor mit Wegdaten
        v = 0;          % Vektor mit Geschwindigkeitsdaten
        nZyklen = 0;    % Anzahl der benoetigten Zyklen
        nZyklenK = 0;
        n = 1;          % Zaehlvariable
        fertig = 0;
    end

    if (enable == 1) || (fertig == 1)
        n = 1;
        startPosition = istPosition;
        % Berechnung der Zeitabschnitte für anfahren, konstant Fahren und bremsen
        tvMax   = 1/aMax * vMax ;       % Zeit bis maximale Geschw.(vMax) erreicht ist
        svMax   = 1/2 * aMax * tvMax^2; % Weg der zurueckgelegt wurde bis tvMax
        tK      = (abs(zielPosition-startPosition) - 2 * svMax) / vMax; % Zeit waehrend konstant gefahren wird
        % Fuer nur Anfahren und Bremsen
        tHalbe = sqrt(2 * 1/aMax * abs(zielPosition-startPosition)/2); % Zeit bis zur halben Strecke

        tBB = zeros(1,nGr);
        tBA = zeros(1,nGr);
        tBK = zeros(1,nGr);
        sA  = zeros(1,nGr);
        vA  = zeros(1,nGr);
        sB  = zeros(1,nGr);
        vB  = zeros(1,nGr);
        sK  = zeros(1,nGr);
        vK  = zeros(1,nGr);
        s   = zeros(1,3*nGr);
        v   = zeros(1,3*nGr);
%         % Nur Anfahren und Bremsen
         if tvMax > tHalbe
            % Beschleunigung/Anfahrt
            nZyklen = ceil(tHalbe/dt);
            nZyklenK = 0;
            if nZyklen > nGr
                nZyklen = nGr;
            elseif nZyklen <= 0
                nZyklen = 1;
            end
            
            tBA(1:nZyklen) = linspace(0,tHalbe,nZyklen);%0:dt:(nZyklen)*dt-dt;

            sA(1:nZyklen) = sign(zielPosition-startPosition) * 1/2 * aMax * tBA(1:nZyklen).^2;
            %sA(sA==0) = [];
            vA(1:nZyklen) = sign(zielPosition-startPosition) *aMax * tBA(1:nZyklen);
            % Bremsen
            tBB(1:nZyklen) = linspace(-tHalbe,0,nZyklen);%-nZyklen*dt+dt:dt:0;
            
            %manchmal klappt das mit dem runden nicht so gut...
            if sA(nZyklen) == 0
                offset = 1;
            else
                offset = 0;
            end
            
            sB(1:nZyklen) = -sign(zielPosition-startPosition) * 1/2 * aMax * tBB(1:nZyklen) .^2 + 2*sA(nZyklen-offset);
            vB(1:nZyklen) = -sign(zielPosition-startPosition) * aMax * tBB(1:nZyklen);
            s(1:2*nZyklen) = [sA(1:nZyklen) sB(1:nZyklen)]+startPosition;
            v(1:2*nZyklen) = [vA(1:nZyklen) vB(1:nZyklen)];
            
        else
            % Beschleunigung/Anfahrt

            nZyklen = ceil((tvMax)/dt);
            nZyklenK = ceil(tK/dt);

            if nZyklen > nGr
                nZyklen = nGr;
            elseif nZyklen <= 0
                nZyklen = 1;
            end
            if nZyklenK > nGr
                nZyklenK = nGr;
            elseif nZyklenK <= 0
                nZyklenK = 1;
            end
            
            tBA(1:nZyklen) = linspace(0,tvMax,nZyklen);%0:dt:(nZyklen)*dt-dt;

            sA(1:nZyklen) = sign(zielPosition-startPosition) * 1/2 * aMax * tBA(1:nZyklen).^2;
            vA(1:nZyklen) = sign(zielPosition-startPosition) * aMax * tBA(1:nZyklen);
            %manchmal klappt das mit dem runden nicht so gut...
            if sA(nZyklen) == 0
                offset = 1;
            else
                offset = 0;
            end
            % Fahrt mit konstanter Geschwindigkeit
            tBK(1:nZyklenK) = linspace(0,tK,nZyklenK);%0:dt:(nZyklenK)*dt-dt;
            vK(1:nZyklenK)   = sign(zielPosition-startPosition) * vMax * ones(1,nZyklenK);
            sK(1:nZyklenK)   = sign(zielPosition-startPosition) * vMax * tBK(1:nZyklenK) + sA(nZyklen-offset);
            if sK(nZyklenK) == 0
                offsetK = 1;
            else
                offsetK = 0;
            end
            % Bremsen
            tBB(1:nZyklen) = linspace(-tvMax,0,nZyklen);%-(nZyklen)*dt+dt:dt:0;

            sB(1:nZyklen) = -sign(zielPosition-startPosition) *  1/2 * aMax * tBB(1:nZyklen).^2 + sA(nZyklen-offset)+sK(nZyklenK-offsetK);
            vB(1:nZyklen) = -sign(zielPosition-startPosition) *  aMax * tBB(1:nZyklen);
            s(1:2*nZyklen+nZyklenK) = [sA(1:nZyklen) sK(1:nZyklenK) sB(1:nZyklen)]+startPosition;
            v(1:2*nZyklen+nZyklenK) = [vA(1:nZyklen) vK(1:nZyklenK) vB(1:nZyklen)];
         end
        firstRun = 0;
    end
    % Ausgabe
    sollPosition = s(n);
    sollGeschwindigkeit = v(n);
    if n < (2*nZyklen+nZyklenK-1)
        n = n + 1;
         fertig = 0;
     elseif nZyklen == nGr || nZyklenK == nGr 
         fertig = 1;
    end

== matlab function Gesamtmodell/Regelung1/Zustandsautomat/KoordonatenTafel1 ==
  data: stationsNr input; zielX output; zielY output; zielPsi output; toleranzStufe output; StationsKoordinaten parameter; enable output; Korrektur input
function [zielX, zielY, zielPsi, toleranzStufe, enable] = koordinaten(stationsNr,StationsKoordinaten,Korrektur)

xBuchtOffset = 10;
% 1 -> genau, 2 -> ungenau
toleranzStufe = 1;
enable = 1;

% Batteriestationen anfahren

if stationsNr == 80
    zielX   = StationsKoordinaten(1,stationsNr);
    zielY   = StationsKoordinaten(2,stationsNr);
    zielPsi = pi;
    return
end

if stationsNr == 90
    zielX   = StationsKoordinaten(1,stationsNr);
    zielY   = StationsKoordinaten(2,stationsNr);
    zielPsi = pi;
    return
end

if stationsNr == 100
    zielX   = StationsKoordinaten(1,stationsNr);
    zielY   = StationsKoordinaten(2,stationsNr);
    zielPsi = pi;
    return
end

if stationsNr == 110
    zielX   = StationsKoordinaten(1,stationsNr);
    zielY   = StationsKoordinaten(2,stationsNr);
    zielPsi = pi;
    return
end

% Warteposition vorne
if mod(stationsNr, 10) == 0 
    toleranzStufe = 2;
    
        % WartePosition 0
        if stationsNr == 0
            %weil Matlab leider nicht von 0 aus zählen kann müssen wir das von
            %Hand abfangen...doofes Matlab
            zielX   = 853;
            zielY   = 2288;
            zielPsi = pi/2;
        else
            zielX   = StationsKoordinaten(1,stationsNr);
            zielY   = StationsKoordinaten(2,stationsNr);
            zielPsi = pi/2;
        end

% Stations-Bucht
elseif 0 < mod(stationsNr, 10) && mod(stationsNr, 10) < 4
    
    zielX   = StationsKoordinaten(1,stationsNr);
    zielY   = StationsKoordinaten(2,stationsNr);
    
    % auf welcher Seite der Station?
    if mod(stationsNr, 20) < 10
        % links
        zielX = zielX + xBuchtOffset+Korrektur *5;
        zielPsi = 0;
    else
        % rechts
        zielX = zielX - xBuchtOffset-Korrektur *5;
        zielPsi = pi;
    end

% Warteposition hinten
elseif mod(stationsNr, 10) == 4
    toleranzStufe = 2;
    
    zielX   = StationsKoordinaten(1,stationsNr);
    zielY   = StationsKoordinaten(2,stationsNr);
    zielPsi = pi/2;

% Warteposition mitte
elseif mod(stationsNr, 10) == 5
    
    zielX   = StationsKoordinaten(1,stationsNr);
    zielY   = StationsKoordinaten(2,stationsNr);
    zielPsi = pi/2;

% Vorposition der Bucht
elseif 5 < mod(stationsNr, 10) && mod(stationsNr, 10) < 9
    
    % auf welcher Seite der Station?
    if mod(stationsNr, 20) < 10
        % links
        zielX   = StationsKoordinaten(1,stationsNr-5) - 100;
        zielY   = StationsKoordinaten(2,stationsNr-5);
        zielPsi = 0;
    else
        % rechts
        zielX   = StationsKoordinaten(1,stationsNr-5) + 100;
        zielY   = StationsKoordinaten(2,stationsNr-5);
        zielPsi = pi;
    end

% eine nicht zugeteilte Stationsnummer wird angefordert
else
    % Roboter anhalten
    enable = 0;

    zielX   = 0;
    zielY   = 0;
    zielPsi = 0;
end

== matlab function Gesamtmodell/Regelung1/Zustandsautomat/zielErreicht ==
  data: roboX input; erreicht output; roboY input; roboPsi input; zielX input; zielY input; zielPsi input; toleranzStufe input
 function erreicht = zielErreicht(roboX, roboY, roboPsi, zielX, zielY, zielPsi, toleranzStufe)

 if( toleranzStufe == 2)
    % ungenau
    transToleranz = 50;
    rotToleranz = pi/2;
 else
    % default = genau
    transToleranz = 15;
    rotToleranz = pi/20;
 end

    erreicht = 0;
    
%     if( TasterGreifer == 1)
%         erreicht = 1;
%         return;
%     end
    
    if( abs(zielX-roboX) > transToleranz)
        return;
    end 
    
    if( abs(zielY-roboY) > transToleranz)
        return;
    end 
       
    if( abs(zielPsi-mod(roboPsi,2*pi)) > rotToleranz)&&( abs(zielPsi+2*pi-mod(roboPsi,2*pi)) > rotToleranz)
        return;
    end   

    erreicht = 1;

end

== matlab function Gesamtmodell/Regelung1/Zustandsregler/Winkelentstoerung ==
  data: Ist input; Soll input; Out output



function Out = Winkel(Ist,Soll)

Ist = mod(Ist, 2*pi);      % Normierung des Ist-Winkels auf das Intervall 0° - 360°
Soll = mod(Soll, 2*pi);    % Normierung des Soll-Winkels auf das Intervall 0° - 360°

if (abs(Soll-Ist) <= pi)   % (1)
    
    Out = Soll - Ist;      % (2)
    
else
    
     if (Soll > Ist)                % (3)
        Out = Soll - Ist - 2*pi;    % (4)
     else
         Out = Soll - Ist + 2*pi;   % (5)
     end
end

% Problem: 
% Beim Durchschreiten der Grenze 0°/360° entsteht ein Sprung in
% der Regeldifferenz beim Winkel, der zu einer unkontrollierten Rotation
% des Robotino führt
% 
% Lösung: 
% Impelementierung einer Fallunterscheidung, die die tatsächliche
% Regeldifferenz unter Berücksichtigung der Grenze 0°/360° ausgibt
% 
% Ansatz: 
% Prüfung, ob die vorgegebene Trajektorie über die kritische Grenze
% führt (1). Führt die Trajektorie über die kritische Grenze, ist
% der Betrag der Differenz zwischen Soll- und Istwert > pi.
% 
% Bei unkritischen Trajektorien wird die Regeldifferenz über die Formel (2)
% zurückgegeben.
%
% Bei kritischen Trajektorien muss zuerst unterschieden werden, in welchem
% Drehsinn die kritische Grenze durchschritten wird (3). Bei positivem
% Drehsinn wird die Differenz nach Formel (4) ermittelt, bei negativem
% Drehsinn wird die Differenz nach Formal (5) ermittelt. 
%
% Die Ausgabe der Regeldifferenz erfolgt immer in Richtung und Betrag, bei
% einem positiven Vorzeichen befindet sich die Sollposition in mathematisch
% positivem Drehsinn, bei einem negativen Vorzeichen befindet sie sich in
% mathematisch negativem Drehsinn. Der Betrag gibt die verbleibene
% Winkeldifferenz zur Sollposition an.

== matlab function Gesamtmodell/Regelung1/enable  ==
  data: BereichsModus input; enableBereich input; enableKamera input; enableBeobachter input; enable output; enableKoord input; enableFlogik input
function enable  = enable(BereichsModus, enableBereich,enableKamera,enableBeobachter,enableKoord,enableFlogik)
    if BereichsModus == 1
        % Fertigungsbereich
        if enableBereich && (enableKamera || enableBeobachter )&& enableKoord && enableFlogik
            enable = 1;
        else 
            enable = 0;
        end
    else
        % Transportbereich
        if enableKamera || enableBeobachter 
            % mindestens kamera oder beobachter muessen funktionieren            
            enable = 1;
        else
            % sonst nix fahren 
            enable = 0;
        end
    end
    
end
